simulink model "Copy_of_NDI"  (R2024b)
settings: Solver=ode4  StartTime=0  StopTime=100  FixedStep=fcs.Ts  RelTol=1e-3
PreLoadFcn:
  | FlightPhase = 'FallingLeaf';
  | % FlightPhase = 'InAir';
  | % FlightPhase = 'TVC_h10000V617alpha2';
  | run('PreLoadFcn.m')
values from neighbouring files (symbols this model uses):
  ControlAllocation = 1    [PreLoadFcn.m]    (also in RunThis_ChiaWei.m = 4; RunThis_LM.m = 4; RunThis_Shao.m; RunThis_james.m = 10)
  DUmax = IN_MAT(k+4,1:m)'    [LP_def.m]    (also in LP_lift.m; LP_sig.m; LP_thrust.m; PreLoadFcn.m = [Aactuator.right_aileron.RateLimitUpper Aactuator.left_ailer)
  DUmin = IN_MAT(k+5,1:m)'    [LP_def.m]    (also in LP_lift.m; LP_sig.m; LP_thrust.m; PreLoadFcn.m = [Aactuator.right_aileron.RateLimitLower Aactuator.left_ailer)
  g = [ 0  0  32.17 ]    [PreLoadFcn.m]
  hground = 0    [PreLoadFcn.m]
  m = m1-1    [CGIwrap.m]    (also in DAISY_CHAINING.m; DA_Allocation.m; LP_BasicSolution.m; LP_def.m)
  Mode_deflection_aileron = 1    [PreLoadFcn.m]    (also in RunThis_ChiaWei.m; RunThis_Shao.m = 0)
  Mode_deflection_elevator = 1    [PreLoadFcn.m]    (also in RunThis_ChiaWei.m; RunThis_Shao.m = 0)
  Mode_deflection_rudder = 1    [PreLoadFcn.m]    (also in RunThis_ChiaWei.m; RunThis_Shao.m = 0)
  Mode_deflection_TVC_y = 1    [PreLoadFcn.m]    (also in RunThis_ChiaWei.m; RunThis_Shao.m = 2)
  Mode_deflection_TVC_z = 1    [PreLoadFcn.m]    (also in RunThis_ChiaWei.m; RunThis_Shao.m = 0)
  N = IN_MAT(k+7:k+15,1:m)    [CGIwrap.m]    (also in DAISY_CHAINING.m; PreLoadFcn.m = [ 1      0     0.25; RunThis_ChiaWei.m = [ 1      0     0.25; RunThis_LM.m = [ 1      0     0.25)
  Ninv_2nozzle = inv(diag([  1/21.5  1/21.5  1/25  1/25  1/30  1/15  1/15  1/15  1/15 ]))    [PreLoadFcn.m]
  Ninv_no_nozzle = diag([    21.5    21.5    25    25    30    0     0     0     0  ])    [PreLoadFcn.m]
  state0 = [IC.npos IC.epos IC.alt IC.q0 IC.q1 IC.q2 IC.q3  IC.p IC.q IC.r IC.alpha IC.beta IC.mu IC.Vt IC.chi IC.gamma]    [PreLoadFcn.m]
  Umax_2nozzle = [Aactuator.right_aileron.AngleLimitUpper  Aactuator.left_aileron.AngleLimitUpper  Aactuator.right_elevator.AngleLimitUpper Aactuator.left_elevator.AngleLimitUpper  Aactuator.rudder.AngleLimitUpper                  Aactuator.TVC_ry.AngleLimitUpper    Aactuator.TVC_rz.AngleLimitUpper  Aactuator.TVC_ly.AngleLimitUpper    Aactuator.TVC_lz.AngleLimitUpper]    [PreLoadFcn.m]
  Umax_no_nozzle = [Aactuator.right_aileron.AngleLimitUpper  Aactuator.left_aileron.AngleLimitUpper  Aactuator.right_elevator.AngleLimitUpper Aactuator.left_elevator.AngleLimitUpper  Aactuator.rudder.AngleLimitUpper                    0 0 0 0]    [PreLoadFcn.m]
  Umin_2nozzle = [Aactuator.aileron.AngleLimitLower  Aactuator.aileron.AngleLimitLower  Aactuator.elevator.AngleLimitLower Aactuator.elevator.AngleLimitLower  Aactuator.rudder.AngleLimitLower                  Aactuator.TVC_ry.AngleLimitLower    Aactuator.TVC_rz.AngleLimitLower Aactuator.TVC_ly.AngleLimitLower    Aactuator.TVC_lz.AngleLimitLower]    [PreLoadFcn.m]
  Umin_no_nozzle = [Aactuator.right_aileron.AngleLimitLower  Aactuator.left_aileron.AngleLimitLower  Aactuator.right_elevator.AngleLimitLower Aactuator.left_elevator.AngleLimitLower  Aactuator.rudder.AngleLimitLower                    0 0 0 0]    [PreLoadFcn.m]
undefined symbols (not defined in the file or in its folder): Aactuator, ac, AeroCoeff, EngineTable, F, fcs, ft, IC, kg, LandingGear, Light, MIL, PIController, s, Sensor, sigbuilder_block, slug, sysID_DAQ, sysID_OBES, WMM2020
libraries: aerolibconvert2 x31, slpidlib x11, simulink x6, sharedutil x4, aerolibatmos2 x3, aerolibwind2 x3, aerolibbdyn x3, aerolibgravity2 x2, sharedtransform x1
(part 14 of 14)

== system Copy_of_NDI/F-16 Vehicle Systems Model/Vehicle/Propulsion(two_nozzles)/Afterburning Turbofan Jet Engine/If Action Subsystem2 ==
  note: Pow_max
      |
      | Pow_min
      |
      | T_idle
      |
      | T_mil
      |
      | T_max
  "input " : Inport
  Action Port : ActionPort  ActionPortLabel=if(u1<50)
  Add : Sum
  Add1 : Sum  Inputs=-+
  Demux : Demux  Outputs=5
  Divide : Product  Inputs=**
  Gain : Gain  Gain=1/50
  Terminator : Terminator
  Terminator1 : Terminator
  T_min : Outport  VectorParamsAs1DForOutWhenUnconnected=off
  wires:
  Demux/3 -> Add1/1, Add/1
  Demux/4 -> Add1/2
  Add1/1 -> Divide/2
  Gain/1 -> Divide/1
  Divide/1 -> Add/2
  Add/1 -> T_min/1
  "input "/1 -> Demux/1
  Demux/2 -> Gain/1
  Demux/5 -> Terminator1/1
  Demux/1 -> Terminator/1

== system Copy_of_NDI/F-16 Vehicle Systems Model/Vehicle/Propulsion(two_nozzles)/Afterburning Turbofan Jet Engine/If Action Subsystem3 ==
  note: Pow_max
      |
      | Pow_min
      |
      | T_idle
      |
      | T_mil
      |
      | T_max
  "input " : Inport
  Action Port : ActionPort  ActionPortLabel=elseif(u1>=50)
  Add : Sum
  Add1 : Sum  Inputs=-+
  Add2 : Sum  Inputs=-+
  Constant : Constant  Value=50
  Demux : Demux  Outputs=5
  Gain : Gain  Gain=1/50
  Product : Product
  Terminator : Terminator
  Terminator1 : Terminator
  T_min : Outport  VectorParamsAs1DForOutWhenUnconnected=off
  wires:
  "input "/1 -> Demux/1
  Demux/4 -> Add/2, Add1/1
  Demux/5 -> Add1/2
  Constant/1 -> Add2/1
  Add2/1 -> Gain/1
  Add1/1 -> Product/2
  Gain/1 -> Product/1
  Product/1 -> Add/1
  Add/1 -> T_min/1
  Demux/3 -> Terminator1/1
  Demux/2 -> Add2/2
  Demux/1 -> Terminator/1

== system Copy_of_NDI/F-16 Vehicle Systems Model/Vehicle/Propulsion(two_nozzles)/Afterburning Turbofan Jet Engine/If Action Subsystem4 ==
  In1 : Inport
  Action Port : ActionPort  ActionPortLabel=if(u3 == u1)
  Out1 : Outport
  wires:
  In1/1 -> Out1/1

== system Copy_of_NDI/F-16 Vehicle Systems Model/Vehicle/Propulsion(two_nozzles)/Afterburning Turbofan Jet Engine/If Action Subsystem5 ==
  In1 : Inport
  Action Port : ActionPort  ActionPortLabel=elseif(u3>u1 & u3<=u2)
  Out1 : Outport
  wires:
  In1/1 -> Out1/1

== system Copy_of_NDI/F-16 Vehicle Systems Model/Vehicle/Propulsion(two_nozzles)/Afterburning Turbofan Jet Engine/If Action Subsystem6 ==
  In1 : Inport
  Action Port : ActionPort  ActionPortLabel=else
  Out1 : Outport
  wires:
  In1/1 -> Out1/1

== system Copy_of_NDI/F-16 Vehicle Systems Model/Vehicle/LandingGear GroundReaction/L Main Gear Geometry Forces and Moments/Calc Gear Force and Pos/Subsystem ==
  note: 地面正向力(慣性座標)
  note: $N=F_{strut} /C_{33}$
  note: $F_{strut} =K{\left(∆z_g^B \right)}+C{\left(∆{\dot{z} }_g^B \right)}$
      | 支柱上的作用力(體座標)
  note: $∆{\dot{z} }_g^B$
  note: 定義：
      | 慣性座標+Z軸朝下
      | 體座標+Z軸朝下
  deltaZgB : Inport
  C33 : Inport  Port=2
  DampingConstant_N/m/sec1 : Gain  Gain=LandingGear.LM.DampingConstant
  NormalForce : Product  Inputs=*/  RndMeth=Zero
  SpringConstant_N/m1 : Gain  Gain=LandingGear.LM.SpringConstant
  Sum2 : Sum
  Xcmpr_prev : Memory  InheritSampleTime=on
  dCompression : Sum  Inputs=+-
  ground only pushes : Saturate  UpperLimit=inf  LowerLimit=0
  reaction : Gain  Gain=-1
  dZ_strut : Outport
  Fn_strut : Outport  Port=2
  wires:
  deltaZgB/1 -> Xcmpr_prev/1, dCompression/1, SpringConstant_N/m1/1, dZ_strut/1
  dCompression/1 -> DampingConstant_N/m/sec1/1
  DampingConstant_N/m/sec1/1 -> Sum2/2
  SpringConstant_N/m1/1 -> Sum2/1
  Sum2/1 -> NormalForce/1  "Fstrut"
  NormalForce/1 -> ground only pushes/1
  ground only pushes/1 -> reaction/1
  reaction/1 -> Fn_strut/1
  Xcmpr_prev/1 -> dCompression/2
  C33/1 -> NormalForce/2

== system Copy_of_NDI/F-16 Vehicle Systems Model/Vehicle/LandingGear GroundReaction/L Main Gear Geometry Forces and Moments/GenerateGroundFM/Forces and distances to LMN ==
  Fb : Inport
  Xg_gnd : Inport  Port=2
  force to moment : Product  Multiplication=Matrix(*)  InputSameDT=on  SaturateOnIntegerOverflow=on  OutDataTypeStr=Inherit: Same as first input
  transpose : Reshape  OutputDimensionality=Row vector (2-D)  OutputDimensions=[1,3]
  transpose1 : Reshape  OutputDimensionality=Column vector (2-D)  OutputDimensions=[1,3]
  LMNe : Outport
  wires:
  Fb/1 -> transpose/1
  transpose/1 -> force to moment/1
  Xg_gnd/1 -> force to moment/2
  force to moment/1 -> transpose1/1
  transpose1/1 -> LMNe/1

== system Copy_of_NDI/F-16 Vehicle Systems Model/Vehicle/LandingGear GroundReaction/L Main Gear Geometry Forces and Moments/GenerateGroundFM/LocMatrix1 ==
  note: 正負號可能相反
  note: $z_g^{B^{\prime } }$
  note: $x_g^B$
  note: ${\left\{\begin{array}{c} L_G =Y_G \cdot z_g^{B^{\prime } } -Z_G \cdot y_g^B \\ M_G =Z_G \cdot x_g^B -X_G \cdot z_g^{B^{\prime } } \\ N_G =X_G \cdot y_g^B -Y_G \cdot x_g^B \end{array}\right)}={\left[\begin{array}{ccc} 0 & z_g^{B^{\prime } } & -y_g^B \\ -z_g^{B^{\prime } } & 0 & x_g^B \\ y_g^B & -x_g^B & 0 \end{array}\right]}{\left[\begin{array}{c} X_G \\ Y_G \\ Z_G \end{array}\right]}={\left[\begin{array}{ccc} A_{11} & A_{12} & A_{13} \\ A_{21} & A_{22} & A_{23} \\ A_{31} & A_{32} & A_{33} \end{array}\right]}{\left[\begin{array}{c} X_G \\ Y_G \\ Z_G \end{array}\right]}$
  note: 詹庭宇:HL-20 example建模正負號有誤
  note: $y_g^B$
  note: $z_g^B$
  XgB : Inport
  ZgB_prime : Inport  Port=2
  Create 3x3 Matrix : sharedutil/Create 3x3 Matrix  aMode=aMode
  Demux2 : Demux  Outputs=3
  Terminator1 : Terminator
  inv1 : Gain  Gain=-1
  inv3 : Gain  Gain=-1
  inv4 : Gain  Gain=-1
  zero1 : Constant  Value=0  SampleTime=0
  zero2 : Constant  Value=0  SampleTime=0
  zero3 : Constant  Value=0  SampleTime=0
  A : Outport
  wires:
  XgB/1 -> Demux2/1
  Create 3x3 Matrix/1 -> A/1
  zero1/1 -> Create 3x3 Matrix/1
  Demux2/3 -> Terminator1/1
  ZgB_prime/1 -> Create 3x3 Matrix/2, inv4/1
  zero2/1 -> Create 3x3 Matrix/5
  zero3/1 -> Create 3x3 Matrix/9
  Demux2/2 -> Create 3x3 Matrix/7, inv1/1
  Demux2/1 -> Create 3x3 Matrix/6, inv3/1
  inv1/1 -> Create 3x3 Matrix/3
  inv4/1 -> Create 3x3 Matrix/4
  inv3/1 -> Create 3x3 Matrix/8

== system Copy_of_NDI/F-16 Vehicle Systems Model/Vehicle/LandingGear GroundReaction/L Main Gear Geometry Forces and Moments/GenerateGroundFM/Rotation Speed(TVC ON) ==
  friction : Inport
  In Bus Element38 : Inport  Port=2  PortName=PlantData  Element=Vt
  Gain1 : Gain  Gain=0.1
  Gain2 : Gain  Gain=0.5
  Switch : Switch  Threshold=180  SaturateOnIntegerOverflow=off  InputSameDT=off
  output : Outport
  wires:
  In Bus Element38/1 -> Switch/2
  friction/1 -> Gain1/1, Gain2/1
  Switch/1 -> output/1
  Gain2/1 -> Switch/3
  Gain1/1 -> Switch/1

== system Copy_of_NDI/F-16 Vehicle Systems Model/Vehicle/LandingGear GroundReaction/Nose Gear Geometry Forces and Moments/Calc Gear Force and Pos/Subsystem ==
  note: 地面正向力(慣性座標)
  note: $N=F_{strut} /C_{33}$
  note: $F_{strut} =K{\left(∆z_g^B \right)}+C{\left(∆{\dot{z} }_g^B \right)}$
      | 支柱上的作用力(體座標)
  note: $∆{\dot{z} }_g^B$
  note: 定義：
      | 慣性座標+Z軸朝下
      | 體座標+Z軸朝下
  deltaZgB : Inport
  C33 : Inport  Port=2
  DampingConstant_N/m/sec1 : Gain  Gain=LandingGear.Nose.DampingConstant
  NormalForce : Product  Inputs=*/  RndMeth=Zero
  SpringConstant_N/m1 : Gain  Gain=LandingGear.Nose.SpringConstant
  Sum2 : Sum
  Xcmpr_prev : Memory  InheritSampleTime=on
  dCompression : Sum  Inputs=+-
  ground only pushes : Saturate  UpperLimit=inf  LowerLimit=0
  reaction : Gain  Gain=-1
  dZ_strut : Outport
  Fn_strut : Outport  Port=2
  wires:
  deltaZgB/1 -> Xcmpr_prev/1, dCompression/1, SpringConstant_N/m1/1, dZ_strut/1
  dCompression/1 -> DampingConstant_N/m/sec1/1
  DampingConstant_N/m/sec1/1 -> Sum2/2
  SpringConstant_N/m1/1 -> Sum2/1
  Sum2/1 -> NormalForce/1  "Fstrut"
  NormalForce/1 -> ground only pushes/1
  ground only pushes/1 -> reaction/1
  reaction/1 -> Fn_strut/1
  Xcmpr_prev/1 -> dCompression/2
  C33/1 -> NormalForce/2

== system Copy_of_NDI/F-16 Vehicle Systems Model/Vehicle/LandingGear GroundReaction/Nose Gear Geometry Forces and Moments/GenerateGroundFM/Forces and distances to LMN ==
  Fb : Inport
  Xg_gnd : Inport  Port=2
  force to moment : Product  Multiplication=Matrix(*)  InputSameDT=on  SaturateOnIntegerOverflow=on  OutDataTypeStr=Inherit: Same as first input
  transpose : Reshape  OutputDimensionality=Row vector (2-D)  OutputDimensions=[1,3]
  transpose1 : Reshape  OutputDimensionality=Column vector (2-D)  OutputDimensions=[1,3]
  LMNe : Outport
  wires:
  Fb/1 -> transpose/1
  transpose/1 -> force to moment/1
  Xg_gnd/1 -> force to moment/2
  force to moment/1 -> transpose1/1
  transpose1/1 -> LMNe/1

== system Copy_of_NDI/F-16 Vehicle Systems Model/Vehicle/LandingGear GroundReaction/Nose Gear Geometry Forces and Moments/GenerateGroundFM/LocMatrix1 ==
  note: 正負號可能相反
  note: $z_g^{B^{\prime } }$
  note: $x_g^B$
  note: ${\left\{\begin{array}{c} L_G =Y_G \cdot z_g^{B^{\prime } } -Z_G \cdot y_g^B \\ M_G =Z_G \cdot x_g^B -X_G \cdot z_g^{B^{\prime } } \\ N_G =X_G \cdot y_g^B -Y_G \cdot x_g^B \end{array}\right)}={\left[\begin{array}{ccc} 0 & z_g^{B^{\prime } } & -y_g^B \\ -z_g^{B^{\prime } } & 0 & x_g^B \\ y_g^B & -x_g^B & 0 \end{array}\right]}{\left[\begin{array}{c} X_G \\ Y_G \\ Z_G \end{array}\right]}={\left[\begin{array}{ccc} A_{11} & A_{12} & A_{13} \\ A_{21} & A_{22} & A_{23} \\ A_{31} & A_{32} & A_{33} \end{array}\right]}{\left[\begin{array}{c} X_G \\ Y_G \\ Z_G \end{array}\right]}$
  note: 詹庭宇:HL-20 example建模正負號有誤
  note: $y_g^B$
  note: $z_g^B$
  XgB : Inport
  ZgB_prime : Inport  Port=2
  Create 3x3 Matrix : sharedutil/Create 3x3 Matrix  aMode=aMode
  Demux2 : Demux  Outputs=3
  Terminator1 : Terminator
  inv1 : Gain  Gain=-1
  inv3 : Gain  Gain=-1
  inv4 : Gain  Gain=-1
  zero1 : Constant  Value=0  SampleTime=0
  zero2 : Constant  Value=0  SampleTime=0
  zero3 : Constant  Value=0  SampleTime=0
  A : Outport
  wires:
  XgB/1 -> Demux2/1
  Create 3x3 Matrix/1 -> A/1
  zero1/1 -> Create 3x3 Matrix/1
  Demux2/3 -> Terminator1/1
  ZgB_prime/1 -> Create 3x3 Matrix/2, inv4/1
  zero2/1 -> Create 3x3 Matrix/5
  zero3/1 -> Create 3x3 Matrix/9
  Demux2/2 -> Create 3x3 Matrix/7, inv1/1
  Demux2/1 -> Create 3x3 Matrix/6, inv3/1
  inv1/1 -> Create 3x3 Matrix/3
  inv4/1 -> Create 3x3 Matrix/4
  inv3/1 -> Create 3x3 Matrix/8

== system Copy_of_NDI/F-16 Vehicle Systems Model/Vehicle/LandingGear GroundReaction/Nose Gear Geometry Forces and Moments/GenerateGroundFM/Rotation Speed(TVC ON) ==
  friction : Inport
  In Bus Element38 : Inport  Port=2  PortName=PlantData  Element=Vt
  Gain1 : Gain  Gain=0.1
  Gain2 : Gain  Gain=0.5
  Switch : Switch  Threshold=180  SaturateOnIntegerOverflow=off  InputSameDT=off
  output : Outport
  wires:
  In Bus Element38/1 -> Switch/2
  friction/1 -> Gain1/1, Gain2/1
  Switch/1 -> output/1
  Gain2/1 -> Switch/3
  Gain1/1 -> Switch/1

== system Copy_of_NDI/F-16 Vehicle Systems Model/Vehicle/LandingGear GroundReaction/R Main Gear Geometry Forces and Moments/Calc Gear Force and Pos/Subsystem ==
  note: 地面正向力(慣性座標)
  note: $N=F_{strut} /C_{33}$
  note: $F_{strut} =K{\left(∆z_g^B \right)}+C{\left(∆{\dot{z} }_g^B \right)}$
      | 支柱上的作用力(體座標)
  note: $∆{\dot{z} }_g^B$
  note: 定義：
      | 慣性座標+Z軸朝下
      | 體座標+Z軸朝下
  deltaZgB : Inport
  C33 : Inport  Port=2
  DampingConstant_N/m/sec1 : Gain  Gain=LandingGear.RM.DampingConstant
  NormalForce : Product  Inputs=*/  RndMeth=Zero
  SpringConstant_N/m1 : Gain  Gain=LandingGear.RM.SpringConstant
  Sum2 : Sum
  Xcmpr_prev : Memory  InheritSampleTime=on
  dCompression : Sum  Inputs=+-
  ground only pushes : Saturate  UpperLimit=inf  LowerLimit=0
  reaction : Gain  Gain=-1
  dZ_strut : Outport
  Fn_strut : Outport  Port=2
  wires:
  deltaZgB/1 -> Xcmpr_prev/1, dCompression/1, SpringConstant_N/m1/1, dZ_strut/1
  dCompression/1 -> DampingConstant_N/m/sec1/1
  DampingConstant_N/m/sec1/1 -> Sum2/2
  SpringConstant_N/m1/1 -> Sum2/1
  Sum2/1 -> NormalForce/1  "Fstrut"
  NormalForce/1 -> ground only pushes/1
  ground only pushes/1 -> reaction/1
  reaction/1 -> Fn_strut/1
  Xcmpr_prev/1 -> dCompression/2
  C33/1 -> NormalForce/2

== system Copy_of_NDI/F-16 Vehicle Systems Model/Vehicle/LandingGear GroundReaction/R Main Gear Geometry Forces and Moments/GenerateGroundFM/Forces and distances to LMN ==
  Fb : Inport
  Xg_gnd : Inport  Port=2
  force to moment : Product  Multiplication=Matrix(*)  InputSameDT=on  SaturateOnIntegerOverflow=on  OutDataTypeStr=Inherit: Same as first input
  transpose : Reshape  OutputDimensionality=Row vector (2-D)  OutputDimensions=[1,3]
  transpose1 : Reshape  OutputDimensionality=Column vector (2-D)  OutputDimensions=[1,3]
  LMNe : Outport
  wires:
  Fb/1 -> transpose/1
  transpose/1 -> force to moment/1
  Xg_gnd/1 -> force to moment/2
  force to moment/1 -> transpose1/1
  transpose1/1 -> LMNe/1

== system Copy_of_NDI/F-16 Vehicle Systems Model/Vehicle/LandingGear GroundReaction/R Main Gear Geometry Forces and Moments/GenerateGroundFM/LocMatrix1 ==
  note: 正負號可能相反
  note: $z_g^{B^{\prime } }$
  note: $x_g^B$
  note: ${\left\{\begin{array}{c} L_G =Y_G \cdot z_g^{B^{\prime } } -Z_G \cdot y_g^B \\ M_G =Z_G \cdot x_g^B -X_G \cdot z_g^{B^{\prime } } \\ N_G =X_G \cdot y_g^B -Y_G \cdot x_g^B \end{array}\right)}={\left[\begin{array}{ccc} 0 & z_g^{B^{\prime } } & -y_g^B \\ -z_g^{B^{\prime } } & 0 & x_g^B \\ y_g^B & -x_g^B & 0 \end{array}\right]}{\left[\begin{array}{c} X_G \\ Y_G \\ Z_G \end{array}\right]}={\left[\begin{array}{ccc} A_{11} & A_{12} & A_{13} \\ A_{21} & A_{22} & A_{23} \\ A_{31} & A_{32} & A_{33} \end{array}\right]}{\left[\begin{array}{c} X_G \\ Y_G \\ Z_G \end{array}\right]}$
  note: 詹庭宇:HL-20 example建模正負號有誤
  note: $y_g^B$
  note: $z_g^B$
  XgB : Inport
  ZgB_prime : Inport  Port=2
  Create 3x3 Matrix : sharedutil/Create 3x3 Matrix  aMode=aMode
  Demux2 : Demux  Outputs=3
  Terminator1 : Terminator
  inv1 : Gain  Gain=-1
  inv3 : Gain  Gain=-1
  inv4 : Gain  Gain=-1
  zero1 : Constant  Value=0  SampleTime=0
  zero2 : Constant  Value=0  SampleTime=0
  zero3 : Constant  Value=0  SampleTime=0
  A : Outport
  wires:
  XgB/1 -> Demux2/1
  Create 3x3 Matrix/1 -> A/1
  zero1/1 -> Create 3x3 Matrix/1
  Demux2/3 -> Terminator1/1
  ZgB_prime/1 -> Create 3x3 Matrix/2, inv4/1
  zero2/1 -> Create 3x3 Matrix/5
  zero3/1 -> Create 3x3 Matrix/9
  Demux2/2 -> Create 3x3 Matrix/7, inv1/1
  Demux2/1 -> Create 3x3 Matrix/6, inv3/1
  inv1/1 -> Create 3x3 Matrix/3
  inv4/1 -> Create 3x3 Matrix/4
  inv3/1 -> Create 3x3 Matrix/8

== system Copy_of_NDI/F-16 Vehicle Systems Model/Vehicle/LandingGear GroundReaction/R Main Gear Geometry Forces and Moments/GenerateGroundFM/Rotation Speed(TVC ON) ==
  friction : Inport
  In Bus Element38 : Inport  Port=2  PortName=PlantData  Element=Vt
  Gain1 : Gain  Gain=0.1
  Gain2 : Gain  Gain=0.5
  Switch : Switch  Threshold=180  SaturateOnIntegerOverflow=off  InputSameDT=off
  output : Outport
  wires:
  In Bus Element38/1 -> Switch/2
  friction/1 -> Gain1/1, Gain2/1
  Switch/1 -> output/1
  Gain2/1 -> Switch/3
  Gain1/1 -> Switch/1

== matlab function Copy_of_NDI/F-16 Vehicle Systems Model/Aerodynamic2/ISP /MATLAB Function ==
  data: h input; ISP_output output
function ISP_output =ISP(h)
%%  Symbol:
% a = Speed of sound.
% C = The temperature in Celsius.
% Cv = Constant volime ; Cv = e(internal energy)/T.
% Cp = Constant pressure ; Cp = h(enthalpy)/T.
% e = Internal energy.
% e_tr = Translational energy.
% e_rot = Rotational energy.
% e_vib = Vibrational energy.
% g = Is the gravitational acceleration at height h above sea level.
% go = Is the standard gravitational acceleration.
% gamma = Define Cp(constant pressure)/Cv(constant volime).
% h = Geometric altitude.
% mu = Coefficient of viscosity.
% P = The standard atmosphere at h.
% re = Is the Earth's mean radius.
% R = The gas constant for air.
% T = Is temperature in K.
% To = Is the sea_level temperature (absolute).
% rho = Density.
%% Gravitational acceleration 
go=9.806645;     % m/s^2
re=6356766;      % m
g=go*(re/(re+h))^2;
%%  Standard Atmosphere and Temperature
if h<11000 %11000m 以下
    P = (1013.25*(1-(2.25577e-5*h))^5.255879)*100 ;%unit Pa
    T = 288.15-((6.5e-3*h)); %unit K
elseif h ==11000
    P = 2.263203776117090e+04; %unit Pa
    T = 216.6500; %unit K
elseif h>11000 && h<20000 
    P = (226.32*exp(-0.000157688*(h-11000)) )*100; %unit Pa
    T = 216.6500; %unit K
elseif h==20000
    P = 5.474893557709153e+03; %unit Pa
    T = 216.6500; %unit K
else
    P = (54.7482*((1+4.61574e-6*(h-20000)))^-34.163215)*100 ; %unit Pa
    T = 216.6500+1e-3*(h-20000);%unit K
end
%%  Density
% The gas constant for air in SI units [(N*m)/(kg*K)].
R=287.0528;
rho=P/(R*T);
%%  Coefficient of viscosity
% Viscosity in SI units [kg/(s*m)].
mu=1.458*(10^-6)*((T^1.5)/(T+110.4));
%%  Speed of sound 
% molecular energy.
e_tr=(3/2)*R*T;
e_rot=R*T;
e_vib=(1/2)*R*T;
if ( T >= 600 ) % when the air temperature reaches 600K or higher .
    e=e_tr+e_rot+e_vib;
    Cv=e/T;
    Cp=(e+R*T)/T;
else
    e=e_tr+e_rot;
    Cv=e/T;
    Cp=(e+R*T)/T;
end
gamma=Cp/Cv;
% Speed of sound .
a=sqrt(gamma*R*T);
%%
ISP_output = [T,a,P,rho,g,mu];

== matlab function Copy_of_NDI/F-16 Vehicle Systems Model/μαβ NDI Controller/attitude NDI ==
  data: y_bar input; p_c output; g2 input; q_c output; r_c output
function [p_c, q_c, r_c] = NDI(y_bar, g2)

u_bar = g2 \ y_bar;
% u_bar =pinv(g_s)*y_bar;     
p_c = u_bar(1);
q_c = u_bar(2);
r_c = u_bar(3);


end

== matlab function Copy_of_NDI/F-16 Vehicle Systems Model/Vehicle/6DOF (Quaternion)/Quateration ==
  data: Q input; phi output; theta output; psi output
function [phi,theta,psi] =Quateration(Q)

q0 = Q(1);
q1 = Q(2);
q2 = Q(3);
q3 = Q(4);

%% phi
phi_a = (2*(q0*q1+q2*q3));
phi_b = (q0.^2-q1.^2-q2.^2+q3.^2);
phi = atan2(phi_a,phi_b);%rad
% if phi>180
%     phi = 360-abs(phi);
% end
%% theta
theta = asin((2*q0*q2)-(2*q3*q1));%rad
% psi = atan((2*(q0*q3+q1*q2))/(q0.^2+q1.^2-q2.^2-q3.^2));%rad
% phi = atan((2*(q0*q1+q2*q3))/(q0.^2-q1.^2-q2.^2+q3.^2));%rad
%% psi
psi_a = (2*(q0*q3+q1*q2));
psi_b = (q0.^2+q1.^2-q2.^2-q3.^2);
psi = atan2(psi_a,psi_b);%rad
% if psi>180
%     psi = 360-abs(psi);
% end
%%
%test q0^2+q1^2+q2^2+Q3^3=1
% test = q0.^2+q1.^2+q2.^2+q3.^2;
% Quater = [phi theta psi test];

% Quater=zeros(1,4);
% Quater(1)= phi;
% Quater(2)= theta;
% Quater(3)= psi;
% Quater(4)= test;
end

== matlab function Copy_of_NDI/Environment/ISP /MATLAB Function ==
  data: h input; ISP_output output
function ISP_output =ISP(h)
%%  Symbol:
% a = Speed of sound.
% C = The temperature in Celsius.
% Cv = Constant volime ; Cv = e(internal energy)/T.
% Cp = Constant pressure ; Cp = h(enthalpy)/T.
% e = Internal energy.
% e_tr = Translational energy.
% e_rot = Rotational energy.
% e_vib = Vibrational energy.
% g = Is the gravitational acceleration at height h above sea level.
% go = Is the standard gravitational acceleration.
% gamma = Define Cp(constant pressure)/Cv(constant volime).
% h = Geometric altitude.
% mu = Coefficient of viscosity.
% P = The standard atmosphere at h.
% re = Is the Earth's mean radius.
% R = The gas constant for air.
% T = Is temperature in K.
% To = Is the sea_level temperature (absolute).
% rho = Density.
%% Gravitational acceleration 
go=9.806645;     % m/s^2
re=6356766;      % m
g=go*(re/(re+h))^2;
%%  Standard Atmosphere and Temperature
if h<11000 %11000m 以下
    P = (1013.25*(1-(2.25577e-5*h))^5.255879)*100 ;%unit Pa
    T = 288.15-((6.5e-3*h)); %unit K
elseif h ==11000
    P = 2.263203776117090e+04; %unit Pa
    T = 216.6500; %unit K
elseif h>11000 && h<20000 
    P = (226.32*exp(-0.000157688*(h-11000)) )*100; %unit Pa
    T = 216.6500; %unit K
elseif h==20000
    P = 5.474893557709153e+03; %unit Pa
    T = 216.6500; %unit K
else
    P = (54.7482*((1+4.61574e-6*(h-20000)))^-34.163215)*100 ; %unit Pa
    T = 216.6500+1e-3*(h-20000);%unit K
end
%%  Density
% The gas constant for air in SI units [(N*m)/(kg*K)].
R=287.0528;
rho=P/(R*T);
%%  Coefficient of viscosity
% Viscosity in SI units [kg/(s*m)].
mu=1.458*(10^-6)*((T^1.5)/(T+110.4));
%%  Speed of sound 
% molecular energy.
e_tr=(3/2)*R*T;
e_rot=R*T;
e_vib=(1/2)*R*T;
if ( T >= 600 ) % when the air temperature reaches 600K or higher .
    e=e_tr+e_rot+e_vib;
    Cv=e/T;
    Cp=(e+R*T)/T;
else
    e=e_tr+e_rot;
    Cv=e/T;
    Cp=(e+R*T)/T;
end
gamma=Cp/Cv;
% Speed of sound .
a=sqrt(gamma*R*T);
%%
ISP_output = [T,a,P,rho,g,mu];

== matlab function Copy_of_NDI/F-16 Vehicle Systems Model/Aerodynamic1/ISP /MATLAB Function ==
  data: h input; ISP_output output
function ISP_output =ISP(h)
%%  Symbol:
% a = Speed of sound.
% C = The temperature in Celsius.
% Cv = Constant volime ; Cv = e(internal energy)/T.
% Cp = Constant pressure ; Cp = h(enthalpy)/T.
% e = Internal energy.
% e_tr = Translational energy.
% e_rot = Rotational energy.
% e_vib = Vibrational energy.
% g = Is the gravitational acceleration at height h above sea level.
% go = Is the standard gravitational acceleration.
% gamma = Define Cp(constant pressure)/Cv(constant volime).
% h = Geometric altitude.
% mu = Coefficient of viscosity.
% P = The standard atmosphere at h.
% re = Is the Earth's mean radius.
% R = The gas constant for air.
% T = Is temperature in K.
% To = Is the sea_level temperature (absolute).
% rho = Density.
%% Gravitational acceleration 
go=9.806645;     % m/s^2
re=6356766;      % m
g=go*(re/(re+h))^2;
%%  Standard Atmosphere and Temperature
if h<11000 %11000m 以下
    P = (1013.25*(1-(2.25577e-5*h))^5.255879)*100 ;%unit Pa
    T = 288.15-((6.5e-3*h)); %unit K
elseif h ==11000
    P = 2.263203776117090e+04; %unit Pa
    T = 216.6500; %unit K
elseif h>11000 && h<20000 
    P = (226.32*exp(-0.000157688*(h-11000)) )*100; %unit Pa
    T = 216.6500; %unit K
elseif h==20000
    P = 5.474893557709153e+03; %unit Pa
    T = 216.6500; %unit K
else
    P = (54.7482*((1+4.61574e-6*(h-20000)))^-34.163215)*100 ; %unit Pa
    T = 216.6500+1e-3*(h-20000);%unit K
end
%%  Density
% The gas constant for air in SI units [(N*m)/(kg*K)].
R=287.0528;
rho=P/(R*T);
%%  Coefficient of viscosity
% Viscosity in SI units [kg/(s*m)].
mu=1.458*(10^-6)*((T^1.5)/(T+110.4));
%%  Speed of sound 
% molecular energy.
e_tr=(3/2)*R*T;
e_rot=R*T;
e_vib=(1/2)*R*T;
if ( T >= 600 ) % when the air temperature reaches 600K or higher .
    e=e_tr+e_rot+e_vib;
    Cv=e/T;
    Cp=(e+R*T)/T;
else
    e=e_tr+e_rot;
    Cv=e/T;
    Cp=(e+R*T)/T;
end
gamma=Cp/Cv;
% Speed of sound .
a=sqrt(gamma*R*T);
%%
ISP_output = [T,a,P,rho,g,mu];

== matlab function Copy_of_NDI/F-16 Vehicle Systems Model/Vehicle/6DOF (Quaternion)/MATLAB Function ==
  data: dxdt output; xu input; Fxyz input; Mxyz input; AeroFM input; Txyz input; LGxyz input; m input; Ix input; Iy input; Iz input; Ixz input; Heng input; g input
function dxdt = odedot_simulink_TVC_final(xu, Fxyz, Mxyz, AeroFM, Txyz,LGxyz,m,Ix,Iy,Iz,Ixz,Heng,g)
%% Define state 
% 用不到
% npos = xu(1);  %(ft)
% epos = xu(2);  %(ft)
% alt  = xu(3);   %(ft)
%---------------------------Quateration-----------------------
q0 = xu(4);
q1 = xu(5);
q2 = xu(6);
q3 = xu(7);
%--------------------------------------------------
% U = xu(8);%(ft/s)
% V = xu(9);%(ft/s)
% W = xu(10);%(ft/s)

% vt = xu(8);%(ft/s)
% alpha = xu(9);%(rad)****
% beta = xu(10);%(rad)****
P = xu(8);%(rad/s)
Q = xu(9);%(rad/s)
R = xu(10);%(rad/s)

alpha = xu(11);
beta = xu(12);
mu = xu(13);
vt = xu(14);
chi = xu(15);
gamma = xu(16);

%-------------------------control----------------------
% 推力
Tx   = Txyz(1);
Ty   = Txyz(2);
Tz   = Txyz(3);
% Mx_T = xu(20);
% My_T = xu(21);
% Mz_T = xu(22);

% 用不到
% T = xu(23);%(lbs)
% el = xu(24);%(deg)
% ail = xu(25);%(deg)
% rud = xu(26);%(deg)
% delta_z = xu(27);%(deg)
% delta_y = xu(28);%(deg)

%% ISP
% qbar = xu(29);
%% Aerodynamic coefficient
% CXT = xu(30);
% CYT = xu(31);
% CZT = xu(32);
% CLT = xu(33);
% CMT = xu(34);
% CNT = xu(35);

% lef = xu(36);%(deg)



%% Dimension Convert
% r2d = 180/pi;    %rad to deg
% d2r = pi/180;    %deg to rad
% m2f = 3.2808399; %meter to ft. Same as m/s to ft/s
% f2m = 0.3048;    %ft to meter. Same as ft/s to m/s
%
% theta = asin((2*q0*q2)-(2*q3*q1));%rad
% psi = atan((2*(q0*q3+q1*q2))/(q0^2+q1^2-q2^2-q3^2));%rad
% phi = atan((2*(q0*q1+q2*q3))/(q0^2-q1^2-q2^2+q3^2));%rad

%% Aircraft parameters
% g = 32.17;       %gravity, ft/s^2
% m  = 636.94;     %mass, slugs
% B  = 30.0;       %span, ft
% S = 300.0;       %planform area, ft^2
% cbar = 11.32;    %mean aero chord, ft
% x_cg_ref = 0.35;     %reference center of gravity as a fraction of cbar
% x_cg = 0.30;      %center of gravity as a fraction of cbar.
% Heng = 0.0;      %turbine momentum along roll axis.

% Ix = 9496.0;     %slug-ft^2
% Iy = 55814.0;    %slug-ft^2
% Iz = 63100.0;    %slug-ft^2
% Ixz = 982.0;     %slug-ft^2
%-------------------------Abbreviation----------------------
sa = sin(alpha);  %sin(alpha)
ca = cos(alpha);  %cos(alpha)
sb = sin(beta);  %sin(beta)
cb = cos(beta);  %cos(beta)
tb = tan(beta);  %tan(beta)
% st = sin(theta);  %cos(beta)
% ct = cos(theta);
% tt = tan(theta);
% sphi = sin(phi);
% cphi = cos(phi);
% spsi = sin(psi);
% cpsi = cos(psi);

% %% Calculate Aerdynamic Coefficients
% % [alpha,beta,ele,ail,rud,lef,tot_V,p,q,r]
% Aero_coe = [alpha*r2d,beta*r2d,el,ail,rud,lef,vt,P,Q,R];       %Simulink type
% [Aerodynamic_coe] = Aerodynamic_coefficient(Aero_coe);   %[Cx_tot Cy_tot Cz_tot Cl_tot Cm_tot Cn_tot];
% %% Calculate ISP
% h = alt*f2m;   %ISP code h is meter! Must changed(alt:feet)
% ISP_output = Standard_Atmosphere1(h); %[T(k),a(m/s),P(Pa),rho(kg/m^3),g(m/s^2),mu]
% % Mach = vt/(ISP_output(2)*m2f);
% qbar = 0.5*( 0.00194032033*ISP_output(4) )*(vt^2);
% % g = ISP_output(5)*m2f
%% Lift Drag Side force
% X = qbar*S*CXT;
% Y = qbar*S*CYT;
% Z = qbar*S*CZT;
X = AeroFM(1);
Y = AeroFM(2);
Z = AeroFM(3);

D = -X*ca*cb - Y*sb - Z*sa*cb;
Y_bar = -X*ca*sb + Y*cb - Z*sa*sb;
L = X*sa - Z*ca;
%% qnorm
QQ = q0^2+q1^2+q2^2+q3^2;
q0 = q0/sqrt(QQ);
q1 = q1/sqrt(QQ);
q2 = q2/sqrt(QQ);
q3 = q3/sqrt(QQ);
%% Equations
U = vt*ca*cb;  % directional velocities.
V = vt*sb;
W = vt*sa*cb;
%% LandingGear force
f = LGxyz(1); % Friction force
N = LGxyz(3); % Normal force
%-------------------------Navigation Equations----------------------
% xdot1 = U*(ct*cpsi) + V*(sphi*cpsi*st - cphi*spsi) +  W*(cphi*st*cpsi + sphi*spsi);%nposdot
% xdot2 = U*(ct*spsi) +  V*(sphi*spsi*st + cphi*cpsi) +  W*(cphi*st*spsi - sphi*cpsi);%eposdot
% xdot3 = -U*st + V*(sphi*ct) + W*(cphi*ct);%altdot
xdot1 = U*(q0*q0+q1*q1-q2*q2-q3*q3) + 2*V*(q1*q2-q0*q3) +  2*W*(q1*q3+q0*q2);%nposdot
xdot2 = 2*U*(q1*q2+q0*q3) +  V*(q0*q0-q1*q1+q2*q2-q3*q3) +  2*W*(q2*q3-q0*q1);%eposdot
xdot3 = 2*U*(q1*q3-q0*q2) + 2*V*(q2*q3+q0*q1) + W*(q0*q0-q1*q1-q2*q2+q3*q3);%altdot
%------------------------- Kinematic Equations----------------------
% xdot4 = P + tt*(Q*sphi + R*cphi);%phidot
% xdot5 = Q*cphi - R*sphi;%theta dot
% xdot6 = (Q*sphi + R*cphi)/ct;%psidot
xdot4 = -0.5*(P*q1+Q*q2+R*q3);
xdot5 = -0.5*(-P*q0-R*q2+Q*q3);
xdot6 = -0.5*(-Q*q0+R*q1-P*q3);
xdot7 = -0.5*(-R*q0-Q*q1+P*q2);
%-------------------------Compute Udot,Vdot, Wdot----------------------
% Udot = R*V - Q*W - g*st + qbar*S*CXT/m + T/m;
% Vdot = P*W - R*U + g*ct*sphi + qbar*S*CYT/m;
% Wdot = Q*U - P*V + g*ct*cphi + qbar*S*CZT/m;

% Udot = R*V - Q*W + 2*g*(q1*q3)-2*g*(q0*q2) + qbar*S*CXT/m + T/m;
% Vdot = P*W - R*U + 2*g*(q2*q3)+2*g*(q0*q1) + qbar*S*CYT/m;
% Wdot = Q*U - P*V + (q0*q0-q1*q1-q2*q2+q3*q3)*g + qbar*S*CZT/m;

% xdot8 = (U*Udot + V*Vdot + W*Wdot)/vt;%vt_dot
% 
% xdot9 = (U*Wdot - W*Udot)/(U*U + W*W);%alpha_dot
% xdot10 = (Vdot*vt - V*xdot8)/(vt*vt*cb);%beta_dot
%-------------------------Compute Pdot, Qdot, and Rdot----------------------
% L_tot = CLT*qbar*S*B;    %get moments from coefficients */
% M_tot = CMT*qbar*S*cbar;
% N_tot = CNT*qbar*S*B;
% L_tot = AeroFM(4);
% M_tot = AeroFM(5);
% N_tot = AeroFM(6);
% 
% Mx = L_tot+Mx_T;
% My = M_tot+My_T;
% Mz = N_tot+Mz_T;

Mx = Mxyz(1);
My = Mxyz(2);
Mz = Mxyz(3);

PQ     = P*Q;
QR     = Q*R;
XXXXX  = Ixz*(Ix-Iy+Iz);
IxzIxz = Ixz^2;
denom  = Ix*Iz - IxzIxz;

xdot8  = (Iz*Mx + Ixz*Mz + XXXXX*PQ + (Iy*Iz-IxzIxz-Iz^2)*QR + Ixz*Q*Heng)/denom;    % Pdot
xdot9  = (My + (Iz-Ix)*P*R + Ixz*(R*R-P*P) - R*Heng)/Iy;                             % Qdot
xdot10 = (Ixz*Mx + Ix*Mz - XXXXX*QR + (-Iy*Ix+IxzIxz+Ix^2)*PQ + Ix*Q*Heng)/denom;    % Rdot
%% alpha beta mu vt chi gamma

xdot11 = Q-tb*(P*ca+R*sa)+ ( ( -L+m*g*cos(gamma)*cos(mu) )+ ( -Tx*sa+Tz*ca ) + ( N*cos(gamma)*cos(mu) ) + ( f*(sin(chi)*sin(mu)+cos(chi)*cos(mu)*sin(gamma)) )) /(m*vt*cb);
% xdot14 = -sa/(vt*cb)*Udot + ca/(vt*cb)*Wdot;

xdot12 = -R*ca + P*sa + ( Y_bar*cb+m*g*cos(gamma)*sin(mu) -Tx*sb*ca + Ty*cb - Tz*sb*sa + N*cos(gamma)*sin(mu) - f*(cos(mu)*sin(chi)-cos(chi)*sin(gamma)*sin(mu)) ) / (m*vt);
% xdot15 = (-sb*ca/vt)*Udot + (cb/vt)*Vdot + (-sb*sa/vt)*Wdot;

xdot13 = ( P*ca+R*sa ) / cb + ( L / ( m*vt ) )*( tan(gamma)*sin(mu)+tb ) + ( (Y_bar + Ty) / (m*vt) )*tan(gamma)*cos(mu)*cb+...
    + (-g/vt)*cos(gamma)*cos(mu)*tb + (Tx*sa - Tz*ca)*( tan(gamma)*sin(mu)+tb ) / (m*vt) - (Tx*ca + Tz*sa)*( tan(gamma)*cos(mu)*sb ) / (m*vt)+...
    - N*tb*cos(gamma)*cos(mu) / (m*vt) - f*( cos(mu)*cos(chi)*sin(gamma)*tb + sin(chi)*tan(gamma) + sin(chi)*tb*sin(mu) ) / (m*vt);

% vt_dot
xdot14 = (-D + Y_bar*sb -m*g*sin(gamma) + Tx*cb*ca + Ty*sb + Tz*cb*sa - N*sin(gamma) + f*cos(chi)*cos(gamma) ) / (m);
% xdot17 = cb*ca*Udot + sb*Vdot + cb*sa*Wdot;

% chi_dot
xdot15 = ( L*sin(mu) + Y_bar*cos(mu)*cb + Tx*( sin(mu)*sa - cos(mu)*sb*ca) + Ty*(cos(mu)*cb) -Tz*( cos(mu)*sb*sa+sin(mu)*ca ) - f*sin(chi) ) / ( m*vt*cos(gamma) );

% gamma_dot
xdot16 = ( L*cos(mu) - Y_bar*sin(mu)*cb - m*g*cos(gamma) + Tx* ( sin(mu)*sb*ca + cos(mu)*sa ) -Ty*(sin(mu)*cb) + Tz*( sin(mu)*sb*sa-cos(mu)*ca ) - N*cos(gamma) - f*cos(chi)*sin(gamma) ) / (m*vt);


%%
dxdt = zeros(16,1);  % 定義局部變數。 The first assignment to a local variable determines its class.
dxdt(1) = xdot1;
dxdt(2) = xdot2;
dxdt(3) = xdot3;
dxdt(4) = xdot4;
dxdt(5) = xdot5;
dxdt(6) = xdot6;
dxdt(7) = xdot7;
dxdt(8) = xdot8;
dxdt(9) = xdot9;
dxdt(10) = xdot10;

dxdt(11) = xdot11;
dxdt(12) = xdot12;
dxdt(13) = xdot13;
dxdt(14) = xdot14;
dxdt(15) = xdot15;
dxdt(16) = xdot16;

end

== matlab function Copy_of_NDI/F-16 Vehicle Systems Model/Vehicle/6DOF (Quaternion)/MATLAB Function2 ==
  data: p input; q input; r input; alpha input; beta input; mu input; vt input; gamma input; an output; ay output; alpha_dot input; beta_dot input; Vt_dot input; g input
function [an,ay] = load_factor(p,q,r,alpha,beta, mu,vt,gamma, alpha_dot, beta_dot, Vt_dot, g)
% p =xu(1);
% q = xu(2);
% r = xu(3);
% alpha =xu(4);
% beta = xu(5);
% mu = xu(6);
% vt = xu(7);
% % chi = xu(8);
% gamma = xu(9);
% g = 32.17;

cb = cos(beta);
ca = cos(alpha);
sb = sin(beta);
sa = sin(alpha);
the = alpha + gamma;
phi = mu;


u = vt*cb*ca;
v = vt*sb;
w = v*cb*sa;

wdot = Vt_dot*cb*ca - alpha_dot*vt*cb*ca + beta_dot*vt*sb*sa;
Vt_dot_s = Vt_dot*sb + beta_dot*vt*cb; 


an = (q*u - p*v + g*cos(the)*cos(phi)-wdot)/g;
ay = (-p*w + r*u - g*cos(the)*sin(phi) + Vt_dot_s)/g;


% anz = an;
% anz = [an ay];
end

== matlab function Copy_of_NDI/F-16 Vehicle Systems Model/pqr NDI Controller/ f1 ==
  data: f1 output size=3; moments input; pqr input; Ix input; Iy input; Iz input; Ixz input
function f1 = NDI_f_fast(moments, pqr,Ix,Iy,Iz,Ixz)
p = pqr(1);
q = pqr(2);
r = pqr(3);
L_hat = moments(1);
M_hat = moments(2);
N_hat = moments(3);

pq = p*q;
qr = q*r;
XXXXX = Ixz*(Ix-Iy+Iz);
IxzIxz = Ixz^2;
denom = Ix*Iz - IxzIxz;

f1 = zeros(3,1);
f1(1) = ( Iz*L_hat + Ixz*N_hat + XXXXX*pq + (Iy*Iz - IxzIxz - Iz^2)*qr ) / denom;
f1(2) = ( M_hat + (Iz-Ix)*p*r + Ixz*(r^2-p^2) ) / Iy;
f1(3) = ( Ixz*L_hat + Ix*N_hat - XXXXX*qr + (-Iy*Ix + IxzIxz + Ix^2)*pq ) / denom;
end

== stateflow chart Copy_of_NDI/F-16 Vehicle Systems Model/Landing_Control/Stateflow ==
  state Three_Wheel
    entry:
    mu=deg2rad(0);
    alpha=deg2rad(0);
    beta=deg2rad(0);
    T=1060;
  state Stop_Sliding
    entry:
    Stop_Simulation();
    state Stop_Simulation [function]
  state Two_Wheel
    entry:
    mu=deg2rad(0);
    alpha=deg2rad(13);
    beta=deg2rad(0);
    T=1060;
  (default) -> Two_Wheel
  Two_Wheel -> Three_Wheel : [Vt<=135]
  Three_Wheel -> Stop_Sliding : [Vt<=0]
  data: T output; Vt input; mu output; alpha output; beta output

== stateflow chart Copy_of_NDI/F-16 Vehicle Systems Model/pqr NDI Controller/Control Allocation/Chart ==
  state DA
  state TakeOff_Landing
  state HighManeuverability
  state Cruise
  state Penetration
  note: 需有一個訊號[被雷達鎖定、飛彈來襲]，
      | 解除突防，跳入直接幾何法(接戰模式)
  (default) -> DA : {CA=4;}
  DA -> (junction 92)
  (junction 110) -> DA
  (junction 92) -> DA [order 3] : [switchhh==0]{CA=4;}
  (junction 92) -> Penetration [order 2] : [switchhh==1]{CA=8;}
  (junction 92) -> (junction 98) [order 1] : [switchhh==0]
  TakeOff_Landing -> (junction 110)
  HighManeuverability -> (junction 110)
  Cruise -> (junction 110)
  Penetration -> (junction 110) : [switchhh==0]
  (junction 98) -> TakeOff_Landing [order 1] : [Vt<300&&altitude<1000]{CA=7;}
  (junction 98) -> (junction 102) [order 2]
  (junction 102) -> HighManeuverability [order 1] : [alpha>35]{CA=9;}
  (junction 102) -> (junction 106) [order 2]
  (junction 106) -> Cruise : [Vt_dot<25&&altitude_dot<25]{CA=6;}
  data: CA output; alpha input; Vt input; altitude input; Vt_dot input; altitude_dot input; switchhh input

== matlab function Copy_of_NDI/F-16 Vehicle Systems Model/pqr NDI Controller/Control Allocation/Pseudo_inverses_ShunYuanChang2019/Control Allocation ==
  data: u_bar output; y_bar input; g1 input; N input
function u_bar = NDI(y_bar, g1, N)
% 聯動式(控制配置)

% 提醒：MATLAB Function模塊的 *.m檔裡面，不能使用disp( ) 打印輸出中文字，不然會回報莫名其妙的錯誤 (port widths or dimensions 錯誤 )
% disp('run Pseudo_inverses_ShunYuanChang2019')

% 權重矩陣N 改由 PreLoadFcn.m 做設定和載入

pseudo_inv_gt_f = pinv(g1*N);
u_bar = N*pseudo_inv_gt_f*y_bar;

% right_aileron  = u_bar(1);
% left_aileron   = u_bar(2)
% right_elevator = u_bar(3);
% left_elevator  = u_bar(4);
% rudder         = u_bar(5);  
% TVC_ry         = u_bar(6);  勁豪跟舜淵的 TVC_Y TVC_Z 定義相反
% TVC_rz         = u_bar(7);
% TVC_ly         = u_bar(6);
% TVC_lz         = u_bar(7);

end
